simulink model "hybrid_linear_e1"  (Simulink 8.1)
settings: Solver=ode45  StartTime=0.0  StopTime=10.0  RelTol=1e-3
values from neighbouring files (symbols this model uses):
  x0 = [1;1]    [optimiser_setup.m]
undefined symbols (not defined in the file or in its folder): A1, A2, newP
libraries: dspmtrx3 x5, simulink x3, Numerical x3, Is_equal_scalar x1, goal x1
settings Model: Creator=dejanira  LastModifiedBy=dejanira
settings DataIOCC: SignalLoggingSaveFormat=Dataset
settings OptimizationCC: ExpressionDepthLimit=128
settings DebuggingCC: FcnCallInpInsideContextMsg=EnableAllAsError
settings GRTTargetCC: CombineOutputUpdateFcns=on  GRTInterface=off

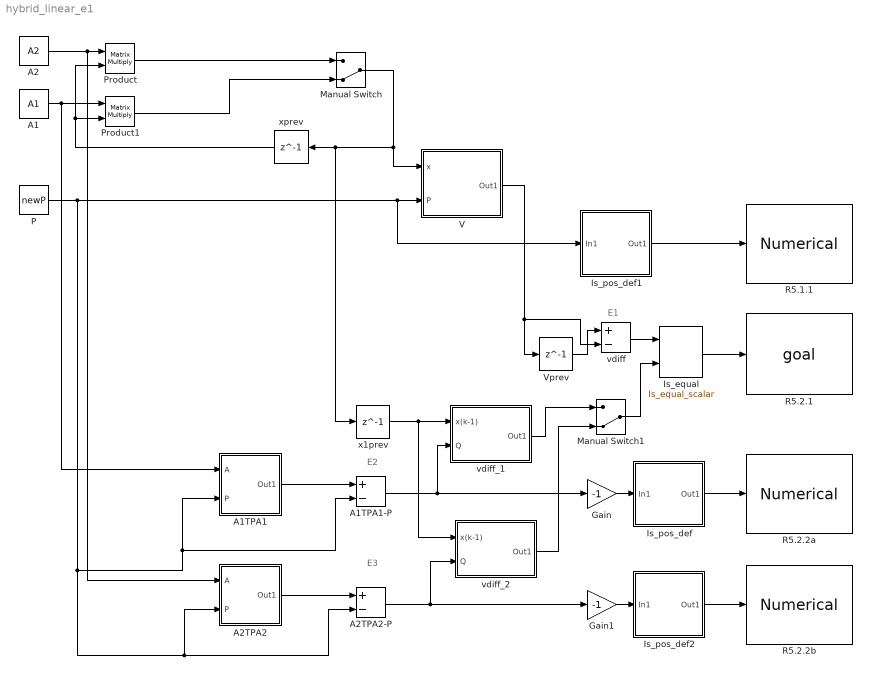
== system hybrid_linear_e1 ==
  note: E1
  note: E2
  note: E3
  A1 : Constant  Value=A1  VectorParams1D=off
  A1TPA1 : Subsystem  mask(Quadratic){}
  A1TPA1-P : Sum  Inputs=+-
  A2 : Constant  Value=A2  VectorParams1D=off
  A2TPA2 : Subsystem  mask(Quadratic){}
  A2TPA2-P : Sum  Inputs=+-
  Gain : Gain  Gain=-1
  Gain1 : Gain  Gain=-1
  Is_equal : Is_equal_scalar/Is_equal_scalar  SystemSampleTime=-1
  Is_pos_def : Subsystem  TreatAsAtomicUnit=on  mask(Is_pos_def){}
      mask Display:
      | port_label('input',1,'matrix')
      | port_label('output',1,'T/F')
  Is_pos_def1 : Subsystem  TreatAsAtomicUnit=on  mask(Is_pos_def){}
      mask Display:
      | port_label('input',1,'matrix')
      | port_label('output',1,'T/F')
  Is_pos_def2 : Subsystem  TreatAsAtomicUnit=on  mask(Is_pos_def){}
      mask Display:
      | port_label('input',1,'matrix')
      | port_label('output',1,'T/F')
  Manual Switch : ManualSwitch  CurrentSetting=0
  Manual Switch1 : ManualSwitch  CurrentSetting=0
  P : Constant  Value=newP
  Product : Product  Multiplication=Matrix(*)
  Product1 : Product  Multiplication=Matrix(*)
  R5.1.1 : Numerical/Numerical  SystemSampleTime=-1
  R5.2.1 : goal/goal  SystemSampleTime=-1
  R5.2.2a : Numerical/Numerical  SystemSampleTime=-1
  R5.2.2b : Numerical/Numerical  SystemSampleTime=-1
  V : Subsystem  mask(Quadratic){}
  Vprev : Delay  DelayLength=1  InitialCondition=x0'*newP*x0  SampleTime=0.1
  vdiff : Sum  Inputs=+-
  vdiff_1 : Subsystem  mask(Quadratic){}
  vdiff_2 : Subsystem  mask(Quadratic){}
  x1prev : Delay  DelayLength=1  InitialCondition=x0
  xprev : Delay  DelayLength=1  InitialCondition=x0
  wires:
  A2/1 -> A2TPA2/1(A), Product/1
  Product/1 -> Manual Switch/1
  A1/1 -> A1TPA1/1(A), Product1/1
  Product1/1 -> Manual Switch/2
  Manual Switch/1 -> x1prev/1, xprev/1, V/1(x)
  A1TPA1-P/1 -> vdiff_1/2(Q), Gain/1
  Is_pos_def/1(Out1) -> R5.2.2a/1
  Gain/1 -> Is_pos_def/1(In1)
  Is_pos_def1/1(Out1) -> R5.1.1/1
  A2TPA2-P/1 -> vdiff_2/2(Q), Gain1/1
  Is_pos_def2/1(Out1) -> R5.2.2b/1
  Gain1/1 -> Is_pos_def2/1(In1)
  P/1 -> A2TPA2-P/2, A2TPA2/2(P), A1TPA1-P/2, A1TPA1/2(P), Is_pos_def1/1(In1), V/2(P)
  vdiff/1 -> Is_equal/1
  Is_equal/1 -> R5.2.1/1
  V/1(Out1) -> vdiff/2, Vprev/1
  A2TPA2/1(Out1) -> A2TPA2-P/1
  A1TPA1/1(Out1) -> A1TPA1-P/1
  Manual Switch1/1 -> Is_equal/2
  x1prev/1 -> vdiff_2/1(x(k-1)), vdiff_1/1(x(k-1))
  vdiff_1/1(Out1) -> Manual Switch1/1
  vdiff_2/1(Out1) -> Manual Switch1/2
  xprev/1 -> Product/2, Product1/2
  Vprev/1 -> vdiff/1

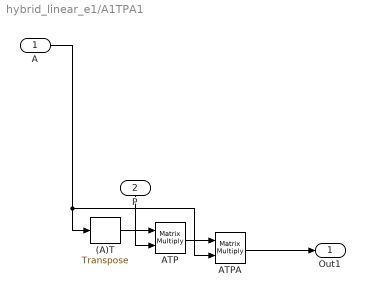
== system hybrid_linear_e1/A1TPA1 ==
  A : Inport
  P : Inport  Port=2
  (A)T : dspmtrx3/Transpose  Hermitian=off  overflowFlag=off
  ATP : Product  Multiplication=Matrix(*)
  ATPA : Product  Multiplication=Matrix(*)
  Out1 : Outport
  wires:
  P/1 -> ATP/2
  (A)T/1 -> ATP/1
  ATPA/1 -> Out1/1
  ATP/1 -> ATPA/1
  A/1 -> (A)T/1, ATPA/2

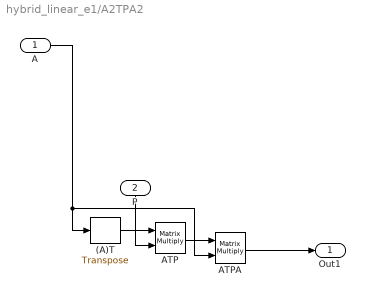
== system hybrid_linear_e1/A2TPA2 ==
  A : Inport
  P : Inport  Port=2
  (A)T : dspmtrx3/Transpose  Hermitian=off  overflowFlag=off
  ATP : Product  Multiplication=Matrix(*)
  ATPA : Product  Multiplication=Matrix(*)
  Out1 : Outport
  wires:
  P/1 -> ATP/2
  (A)T/1 -> ATP/1
  ATPA/1 -> Out1/1
  ATP/1 -> ATPA/1
  A/1 -> (A)T/1, ATPA/2

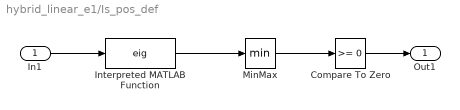
== system hybrid_linear_e1/Is_pos_def ==
  In1 : Inport
  Compare To Zero : simulink/Logic and Bit Operations/Compare To Zero  relop=>=  OutDataTypeStr=boolean
  Interpreted MATLAB Function : MATLABFcn  MATLABFcn=eig
  MinMax : MinMax
  Out1 : Outport
  wires:
  Interpreted MATLAB Function/1 -> MinMax/1
  Compare To Zero/1 -> Out1/1
  In1/1 -> Interpreted MATLAB Function/1
  MinMax/1 -> Compare To Zero/1

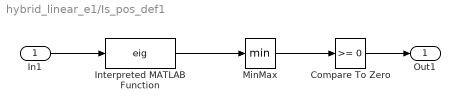
== system hybrid_linear_e1/Is_pos_def1 ==
  In1 : Inport
  Compare To Zero : simulink/Logic and Bit Operations/Compare To Zero  relop=>=  OutDataTypeStr=boolean
  Interpreted MATLAB Function : MATLABFcn  MATLABFcn=eig
  MinMax : MinMax
  Out1 : Outport
  wires:
  Interpreted MATLAB Function/1 -> MinMax/1
  Compare To Zero/1 -> Out1/1
  In1/1 -> Interpreted MATLAB Function/1
  MinMax/1 -> Compare To Zero/1

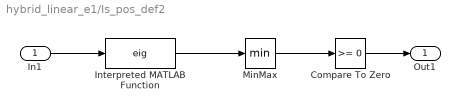
== system hybrid_linear_e1/Is_pos_def2 ==
  In1 : Inport
  Compare To Zero : simulink/Logic and Bit Operations/Compare To Zero  relop=>=  OutDataTypeStr=boolean
  Interpreted MATLAB Function : MATLABFcn  MATLABFcn=eig
  MinMax : MinMax
  Out1 : Outport
  wires:
  Interpreted MATLAB Function/1 -> MinMax/1
  Compare To Zero/1 -> Out1/1
  In1/1 -> Interpreted MATLAB Function/1
  MinMax/1 -> Compare To Zero/1

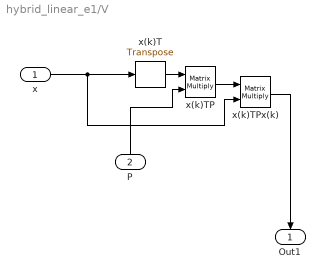
== system hybrid_linear_e1/V ==
  x : Inport
  P : Inport  Port=2
  x(k)T : dspmtrx3/Transpose  Hermitian=off  overflowFlag=off
  x(k)TP : Product  Multiplication=Matrix(*)
  x(k)TPx(k) : Product  Multiplication=Matrix(*)
  Out1 : Outport
  wires:
  x(k)T/1 -> x(k)TP/1
  x(k)TPx(k)/1 -> Out1/1
  P/1 -> x(k)TP/2
  x(k)TP/1 -> x(k)TPx(k)/1
  x/1 -> x(k)TPx(k)/2, x(k)T/1

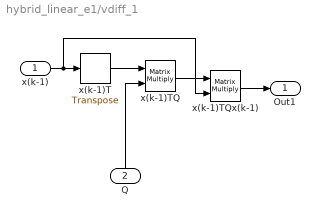
== system hybrid_linear_e1/vdiff_1 ==
  x(k-1) : Inport
  Q : Inport  Port=2
  x(k-1)T : dspmtrx3/Transpose  Hermitian=off  overflowFlag=off
  x(k-1)TQ : Product  Multiplication=Matrix(*)
  x(k-1)TQx(k-1) : Product  Multiplication=Matrix(*)
  Out1 : Outport
  wires:
  Q/1 -> x(k-1)TQ/2
  x(k-1)TQ/1 -> x(k-1)TQx(k-1)/1
  x(k-1)TQx(k-1)/1 -> Out1/1
  x(k-1)T/1 -> x(k-1)TQ/1
  x(k-1)/1 -> x(k-1)TQx(k-1)/2, x(k-1)T/1

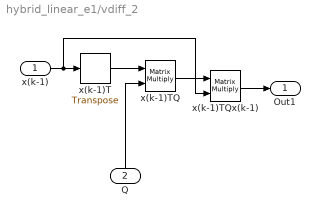
== system hybrid_linear_e1/vdiff_2 ==
  x(k-1) : Inport
  Q : Inport  Port=2
  x(k-1)T : dspmtrx3/Transpose  Hermitian=off  overflowFlag=off
  x(k-1)TQ : Product  Multiplication=Matrix(*)
  x(k-1)TQx(k-1) : Product  Multiplication=Matrix(*)
  Out1 : Outport
  wires:
  Q/1 -> x(k-1)TQ/2
  x(k-1)TQ/1 -> x(k-1)TQx(k-1)/1
  x(k-1)TQx(k-1)/1 -> Out1/1
  x(k-1)T/1 -> x(k-1)TQ/1
  x(k-1)/1 -> x(k-1)TQx(k-1)/2, x(k-1)T/1
